simulink model "feedback_lin_p_with_noise_realistic"  (R2023a)
settings: Solver=ode4  StartTime=0.0  StopTime=10  FixedStep=0.001  RelTol=1e-3
InitFcn:
  | Init_control;
values from neighbouring files (symbols this model uses):
  ModelInit_AngEuler = [0, 0, 0]    [Init_control.m]
  ModelInit_PosE = [0, 0, 0]    [Init_control.m]
  ModelInit_Rads = 0    [Init_control.m]
  ModelInit_RateB = [0, 0, 0]    [Init_control.m]
  ModelInit_VelB = [0, 0, 0]    [Init_control.m]
  P = 0.5 * eye(6)    [Init_control.m]
  Ts = 0.002    [Init_control.m]
undefined symbols (not defined in the file or in its folder): lincontroller, ModelParam_envGravityAcc, ModelParam_motorCr, ModelParam_motorJm, ModelParam_motorT, ModelParam_motorWb, ModelParam_rotorCm, ModelParam_rotorCt, ModelParam_uavCCm, ModelParam_uavCd, ModelParam_uavJ, ModelParam_uavMass, ModelParam_uavR, quadParams
libraries: simulink x2, sharedutil x2
settings Model: Creator=wsh  LastModifiedBy=matte
settings SolverCC: AlgebraicLoopSolver=TrustRegion
settings DataIOCC: ReturnWorkspaceOutputs=off
settings DebuggingCC: UnconnectedInputMsg=warning  UnconnectedOutputMsg=warning  UnconnectedLineMsg=warning  BusObjectLabelMismatch=error  ArithmeticOperatorsInVariantConditions=warning
settings ModelReferenceCC: EnableRefExpFcnMdlSchedulingChecks=on
settings SFSimCC: SimUseLocalCustomCode=off  CustomCodeUndefinedFunction=UseInterfaceOnly
settings RTWCC: RTWUseLocalCustomCode=off
settings CodeAppCC: StateflowObjectComments=on

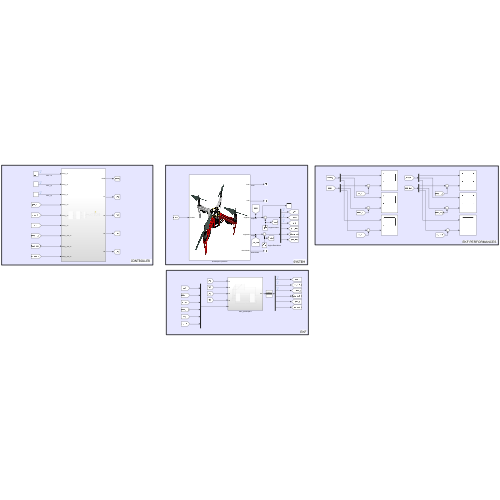
[thumbnail: Simulink's stored preview of the top-level diagram]
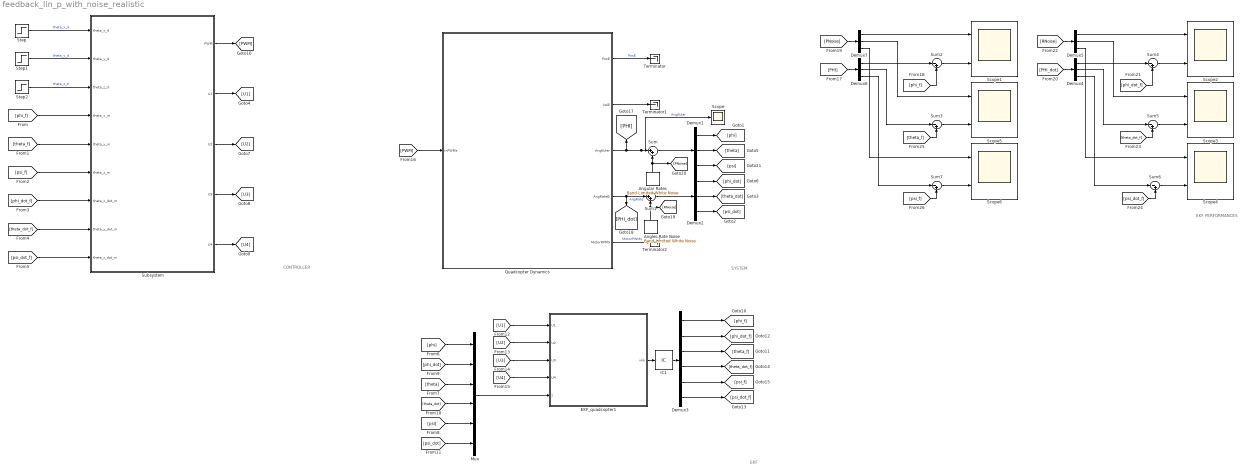
== system feedback_lin_p_with_noise_realistic ==
  note: CONTROLLER
  note: SYSTEM
  note: EKF
  note: EKF PERFORMANCES
  "Angles Rate Noise " : simulink/Sources/Band-Limited White Noise  Cov=[2.782739102258347e-06;2.718240466492716e-06;2.976654513986432e-06]  Ts=Ts  seed=[23341]
  Angular Rates : simulink/Sources/Band-Limited White Noise  Cov=[1.936548166270313e-08;1.809123162388460e-08;5.587443411059212e-06]  Ts=Ts  seed=[23341]
  Demux{1..2,4..7} (6 alike) : Demux  Outputs=3
  Demux3 : Demux  Outputs=6
  EKF_quadcopter1 : Subsystem
  IC1 : InitialCondition  Value=[0;0;0;0;0;0]
  Mux : Mux  Inputs=6
  Quadcopter Dynamics : Subsystem
      mask Display: image('./icon/F450.png');
  Scope : Scope
  Scope{1..6} (6 alike) : Scope  NumInputPorts=2
  Step : Step  After=0.25  SampleTime=0
  Step1 : Step  After=0.5  SampleTime=0
  Step2 : Step  After=0  SampleTime=0
  Subsystem : Subsystem
  Sum : Sum  Inputs=|++
  Sum1 : Sum  Inputs=|++
  Sum{2..7} (6 alike) : Sum  Inputs=|-+
  Terminator : Terminator
  Terminator1 : Terminator
  Terminator2 : Terminator
  wires:
  Step/1 -> Subsystem/1(theta_x_d)  "theta_x_d"
  Step1/1 -> Subsystem/2(theta_y_d)  "theta_y_d"
  Step2/1 -> Subsystem/3(theta_z_d)  "theta_z_d"
  [phi_f] -> Subsystem/4(theta_x_m)
  [theta_f] -> Subsystem/5(theta_y_m)
  [psi_f] -> Subsystem/6(theta_z_m)
  [phi_dot_f] -> Subsystem/7(theta_x_dot_m)
  [theta_dot_f] -> Subsystem/8(theta_y_dot_m)
  [psi_dot_f] -> Subsystem/9(theta_z_dot_m)
  Subsystem/2(U1) -> [U1]
  Subsystem/3(U2) -> [U2]
  Subsystem/4(U3) -> [U3]
  Subsystem/5(U4) -> [U4]
  Subsystem/1(PWM) -> [PWM]
  Demux5/3 -> Scope4/1
  [theta_dot_f] -> Sum5/2
  Demux5/2 -> Scope3/1
  Sum6/1 -> Scope4/2
  [PHI_dot] -> Demux4/1
  Demux4/1 -> Sum4/1
  Demux7/3 -> Scope6/1
  Demux4/2 -> Sum5/1
  Demux6/3 -> Sum7/1
  Demux6/2 -> Sum3/1
  [psi_f] -> Sum7/2
  [PNoise] -> Demux7/1
  Demux7/2 -> Scope5/1
  Sum3/1 -> Scope5/2
  [phi_f] -> Sum2/2
  Demux4/3 -> Sum6/1
  Demux7/1 -> Scope1/1
  Quadcopter Dynamics/4(AngRateB) -> Sum1/1, [PHI_dot]  "AngRate"
  [PHI] -> Demux6/1
  Demux3/2 -> [phi_dot_f]
  Quadcopter Dynamics/5(MotorRPMS) -> Terminator2/1  "MotorPWMs"
  Mux/1 -> EKF_quadcopter1/5(z)
  [psi_dot] -> Mux/6
  [U1] -> EKF_quadcopter1/1(U1)
  Sum2/1 -> Scope1/2
  [phi] -> Mux/1
  Demux6/1 -> Sum2/1
  [U2] -> EKF_quadcopter1/2(U2)
  [RNoise] -> Demux5/1
  Demux2/2 -> [theta_dot]
  [theta] -> Mux/3
  [psi] -> Mux/5
  Sum1/1 -> Demux2/1
  [phi_dot] -> Mux/2
  Angular Rates/1 -> [PNoise], Sum/2
  Demux2/1 -> [phi_dot]
  [U3] -> EKF_quadcopter1/3(U3)
  [theta_f] -> Sum3/2
  Demux1/3 -> [psi]
  [theta_dot] -> Mux/4
  [phi_dot_f] -> Sum4/2
  Sum/1 -> Demux1/1
  IC1/1 -> Demux3/1
  Demux3/3 -> [theta_f]
  Sum4/1 -> Scope2/2
  Demux3/5 -> [psi_f]
  Quadcopter Dynamics/1(PosE) -> Terminator/1  "PosE"
  Demux3/4 -> [theta_dot_f]
  Demux1/2 -> [theta]
  Demux2/3 -> [psi_dot]
  Demux1/1 -> [phi]
  Quadcopter Dynamics/2(VelE) -> Terminator1/1
  Quadcopter Dynamics/3(AngEuler) -> Scope/1, Sum/1, [PHI]  "AngEular"
  [U4] -> EKF_quadcopter1/4(U4)
  Demux3/6 -> [psi_dot_f]
  Sum5/1 -> Scope3/2
  "Angles Rate Noise "/1 -> [RNoise], Sum1/2
  Demux5/1 -> Scope2/1
  [psi_dot_f] -> Sum6/2
  Demux3/1 -> [phi_f]
  [PWM] -> Quadcopter Dynamics/1(inPWMs)
  Sum7/1 -> Scope6/2
  EKF_quadcopter1/1(xkk) -> IC1/1

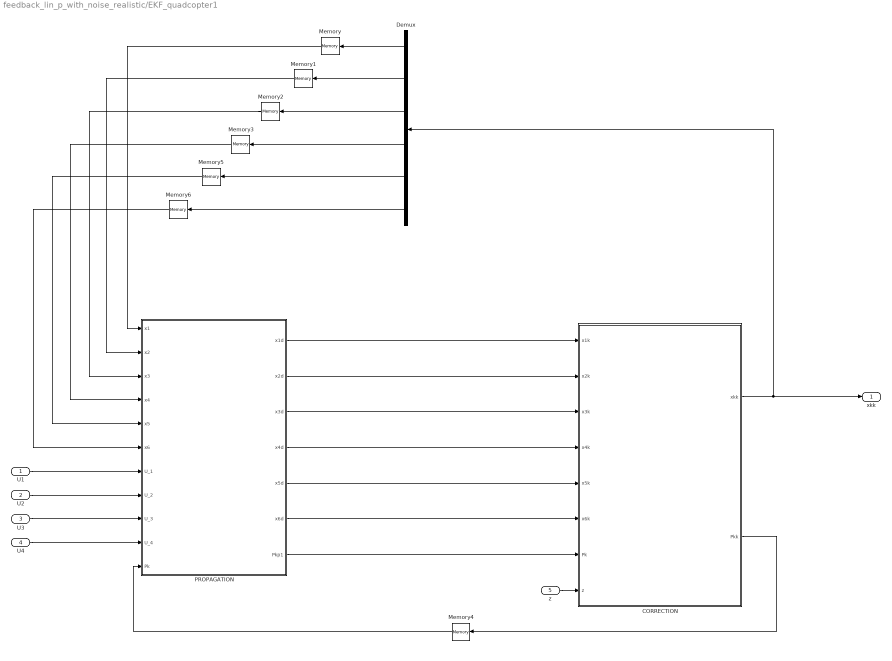
== system feedback_lin_p_with_noise_realistic/EKF_quadcopter1 ==
  U1 : Inport
  U2 : Inport  Port=2
  U3 : Inport  Port=3
  U4 : Inport  Port=4
  z : Inport  Port=5
  CORRECTION : MATLAB Function  TreatAsAtomicUnit=on
  Demux : Demux  Outputs=6
  Memory{,1..3,5..6} (6 alike) : Memory
  Memory4 : Memory  InitialCondition=P
  PROPAGATION : MATLAB Function  TreatAsAtomicUnit=on
  xkk : Outport
  wires:
  PROPAGATION/1(x1d) -> CORRECTION/1(x1k)
  PROPAGATION/2(x2d) -> CORRECTION/2(x2k)
  PROPAGATION/3(x3d) -> CORRECTION/3(x3k)
  PROPAGATION/4(x4d) -> CORRECTION/4(x4k)
  Memory4/1 -> PROPAGATION/11(Pk)
  U1/1 -> PROPAGATION/7(U_1)
  U2/1 -> PROPAGATION/8(U_2)
  U3/1 -> PROPAGATION/9(U_3)
  U4/1 -> PROPAGATION/10(U_4)
  PROPAGATION/7(Pkp1) -> CORRECTION/7(Pk)
  CORRECTION/2(Pkk) -> Memory4/1
  z/1 -> CORRECTION/8(z)
  Demux/1 -> Memory/1
  Demux/2 -> Memory1/1
  Demux/3 -> Memory2/1
  Demux/4 -> Memory3/1
  CORRECTION/1(xkk) -> Demux/1, xkk/1
  Memory/1 -> PROPAGATION/1(x1)
  Memory1/1 -> PROPAGATION/2(x2)
  Memory2/1 -> PROPAGATION/3(x3)
  Memory3/1 -> PROPAGATION/4(x4)
  PROPAGATION/6(x6d) -> CORRECTION/6(x6k)
  PROPAGATION/5(x5d) -> CORRECTION/5(x5k)
  Demux/5 -> Memory5/1
  Memory5/1 -> PROPAGATION/5(x5)
  Demux/6 -> Memory6/1
  Memory6/1 -> PROPAGATION/6(x6)

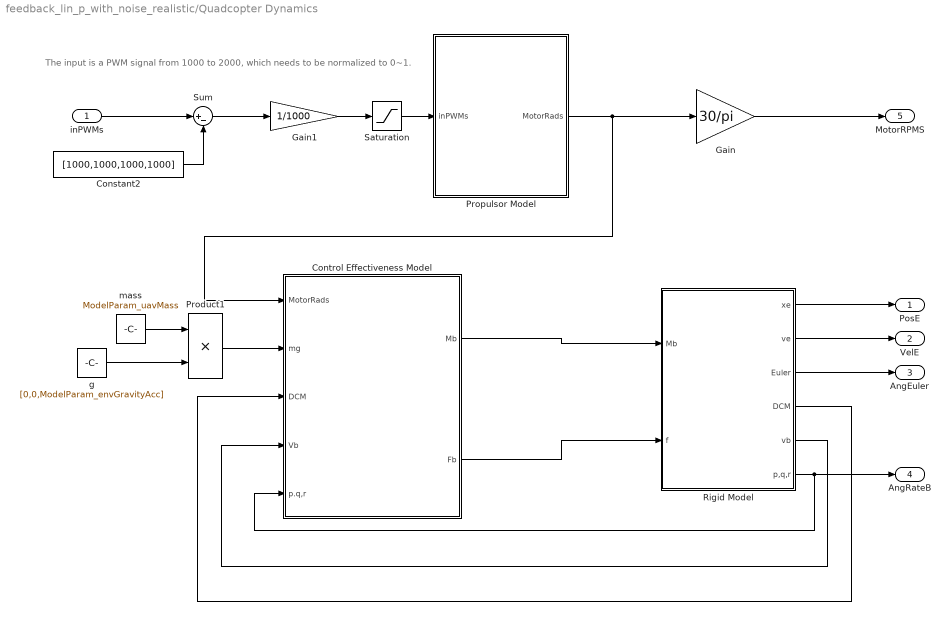
== system feedback_lin_p_with_noise_realistic/Quadcopter Dynamics ==
  note: The input is a PWM signal from 1000 to 2000,
      | which needs to be normalized to 0~1.
  inPWMs : Inport
  Constant2 : Constant  Value=[1000,1000,1000,1000]
  Control Effectiveness Model : Subsystem
  Gain : Gain  Gain=30/pi
  Gain1 : Gain  Gain=1/1000
  Product1 : Product
  Propulsor Model : Subsystem
  Rigid Model : Subsystem
  Saturation : Saturate  UpperLimit=1  LowerLimit=0
  Sum : Sum  Inputs=|+-
  g : Constant  Value=[0,0,ModelParam_envGravityAcc]
  mass : Constant  Value=ModelParam_uavMass
  PosE : Outport  VectorParamsAs1DForOutWhenUnconnected=off
  VelE : Outport  Port=2  VectorParamsAs1DForOutWhenUnconnected=off
  AngEuler : Outport  Port=3  VectorParamsAs1DForOutWhenUnconnected=off
  AngRateB : Outport  Port=4  VectorParamsAs1DForOutWhenUnconnected=off
  MotorRPMS : Outport  Port=5  VectorParamsAs1DForOutWhenUnconnected=off
  wires:
  Saturation/1 -> Propulsor Model/1(inPWMs)
  Rigid Model/6("p,q,r ") -> Control Effectiveness Model/5(p.q,r), AngRateB/1
  mass/1 -> Product1/1
  Rigid Model/4(DCM) -> Control Effectiveness Model/3(DCM)
  Propulsor Model/1(MotorRads) -> Gain/1, Control Effectiveness Model/1(MotorRads)
  Gain1/1 -> Saturation/1
  Rigid Model/2(ve) -> VelE/1
  Sum/1 -> Gain1/1
  Product1/1 -> Control Effectiveness Model/2(mg)
  Rigid Model/5("vb ") -> Control Effectiveness Model/4(Vb)
  Rigid Model/1("xe ") -> PosE/1
  Rigid Model/3(Euler) -> AngEuler/1
  Control Effectiveness Model/1(Mb) -> Rigid Model/1(Mb)
  inPWMs/1 -> Sum/1
  Control Effectiveness Model/2(Fb) -> Rigid Model/2(f)
  Constant2/1 -> Sum/2
  g/1 -> Product1/2
  Gain/1 -> MotorRPMS/1

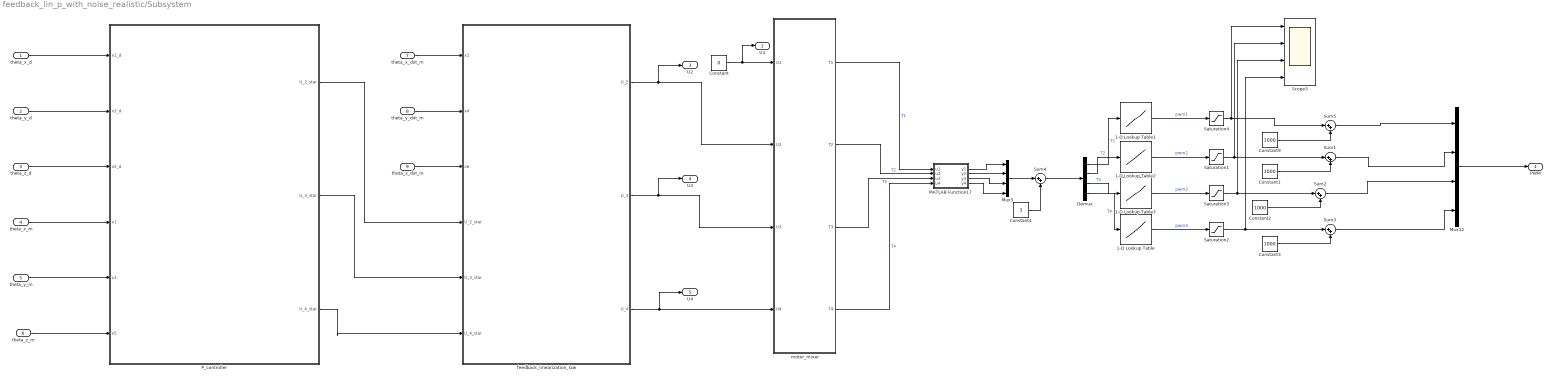
== system feedback_lin_p_with_noise_realistic/Subsystem ==
  theta_x_d : Inport
  theta_y_d : Inport  Port=2
  theta_z_d : Inport  Port=3
  theta_x_m : Inport  Port=4
  theta_y_m : Inport  Port=5
  theta_z_m : Inport  Port=6
  theta_x_dot_m : Inport  Port=7
  theta_y_dot_m : Inport  Port=8
  theta_z_dot_m : Inport  Port=9
  1-D Lookup Table : Lookup_n-D  NumberOfTableDimensions=1  BreakpointsForDimension1=[0;0.06477642396;0.16;0.63;2.44;4.43;6.92;8.77;10.52;11.63;12.03;12.09;12.091;12.092;12.093;12.094;12.095;12.096;12.097;12.098;12.099]  Table=[0;50;100;150;200;250;300;350;400;450;500;550;600;650;700;750;800;850;900;950;1000]  InternalRulePriority=Speed  RndMeth=Simplest
  1-D Lookup Table1 : Lookup_n-D  NumberOfTableDimensions=1  BreakpointsForDimension1=[0;0.02;0.06;0.29;0.73;1.07;1.88;2.91;4;5.06;6.71;7.86;9.41;10.86;11.45;11.82;12.07;12.31;12.52;12.74;12.75]  Table=[0;50;100;150;200;250;300;350;400;450;500;550;600;650;700;750;800;850;900;950;1000]  InternalRulePriority=Speed  RndMeth=Simplest
  1-D Lookup Table2 : Lookup_n-D  NumberOfTableDimensions=1  BreakpointsForDimension1=[0;0.05;0.39;1.67;3.19;5.57;8.07;10.01;10.71;11.06;11.42;11.53;11.55;11.551;11.552;11.553;11.554;11.555;11.556;11.557;11.558]  Table=[0;50;100;150;200;250;300;350;400;450;500;550;600;650;700;750;800;850;900;950;1000]  InternalRulePriority=Speed  RndMeth=Simplest
  1-D Lookup Table3 : Lookup_n-D  NumberOfTableDimensions=1  BreakpointsForDimension1=[0;0.06;0.23;0.89;2.47;3.9;5.86;7.81;9.42;10.12;10.6;11.01;11.34;11.39;11.391;11.392;11.393;11.394;11.395;11.396;11.397]  Table=[0;50;100;150;200;250;300;350;400;450;500;550;600;650;700;750;800;850;900;950;1000]  InternalRulePriority=Speed  RndMeth=Simplest
  Constant : Constant  Value=0
  Constant{1..3,9} (4 alike) : Constant  Value=1000  SampleTime=-1
  Constant4 : Constant  Value=3
  Demux : Demux
  MATLAB Function17 : MATLAB Function  TreatAsAtomicUnit=on
  Mux12 : Mux
  Mux5 : Mux
  P_controller : MATLAB Function  TreatAsAtomicUnit=on
  Saturation{1..4} (4 alike) : Saturate  UpperLimit=1000  LowerLimit=0
  Scope3 : Scope  NumInputPorts=4
  Sum{1..5} (5 alike) : Sum  Inputs=|++
  feedback_linearization_law : MATLAB Function  TreatAsAtomicUnit=on
  motor_mixer : MATLAB Function  SystemSampleTime=0.004
  PWM : Outport  VectorParamsAs1DForOutWhenUnconnected=off
  U1 : Outport  Port=2
  U2 : Outport  Port=3
  U3 : Outport  Port=4
  U4 : Outport  Port=5
  wires:
  theta_x_d/1 -> P_controller/1(x1_d)
  theta_y_d/1 -> P_controller/2(x3_d)
  theta_z_d/1 -> P_controller/3(x5_d)
  theta_x_m/1 -> P_controller/4(x1)
  theta_y_m/1 -> P_controller/5(x3)
  theta_z_m/1 -> P_controller/6(x5)
  Mux12/1 -> PWM/1
  motor_mixer/4(T4) -> MATLAB Function17/4(u4)  "T4"
  1-D Lookup Table3/1 -> Saturation3/1  "pwm3"
  motor_mixer/1(T1) -> MATLAB Function17/1(u1)  "T1"
  motor_mixer/3(T3) -> MATLAB Function17/3(u3)  "T3"
  1-D Lookup Table2/1 -> Saturation1/1  "pwm2"
  1-D Lookup Table1/1 -> Saturation4/1  "pwm1"
  motor_mixer/2(T2) -> MATLAB Function17/2(u2)  "T2"
  Sum5/1 -> Mux12/1
  Saturation4/1 -> Scope3/1, Sum5/1
  Constant9/1 -> Sum5/2
  1-D Lookup Table/1 -> Saturation2/1  "pwm4"
  Saturation1/1 -> Scope3/2, Sum1/1
  Sum1/1 -> Mux12/2
  Constant1/1 -> Sum1/2
  Saturation3/1 -> Scope3/3, Sum2/1
  Sum2/1 -> Mux12/3
  Constant2/1 -> Sum2/2
  Saturation2/1 -> Scope3/4, Sum3/1
  Sum3/1 -> Mux12/4
  Constant3/1 -> Sum3/2
  P_controller/1(U_2_star) -> feedback_linearization_law/4(U_2_star)
  Constant4/1 -> Sum4/2
  Demux/3 -> 1-D Lookup Table3/1  "T3"
  Sum4/1 -> Demux/1
  Mux5/1 -> Sum4/1
  MATLAB Function17/3(y3) -> Mux5/3
  MATLAB Function17/1(y1) -> Mux5/1
  MATLAB Function17/4(y4) -> Mux5/4
  Demux/4 -> 1-D Lookup Table/1  "T4"
  MATLAB Function17/2(y2) -> Mux5/2
  Demux/2 -> 1-D Lookup Table2/1  "T2"
  Demux/1 -> 1-D Lookup Table1/1  "T1"
  feedback_linearization_law/1(U_2) -> U2/1, motor_mixer/2(U2)
  feedback_linearization_law/2(U_3) -> U3/1, motor_mixer/3(U3)
  feedback_linearization_law/3(U_4) -> U4/1, motor_mixer/4(U4)
  P_controller/2(U_3_star) -> feedback_linearization_law/5(U_3_star)
  P_controller/3(U_4_star) -> feedback_linearization_law/6(U_4_star)
  Constant/1 -> U1/1, motor_mixer/1(U1)
  theta_x_dot_m/1 -> feedback_linearization_law/1(x2)
  theta_y_dot_m/1 -> feedback_linearization_law/2(x4)
  theta_z_dot_m/1 -> feedback_linearization_law/3(x6)

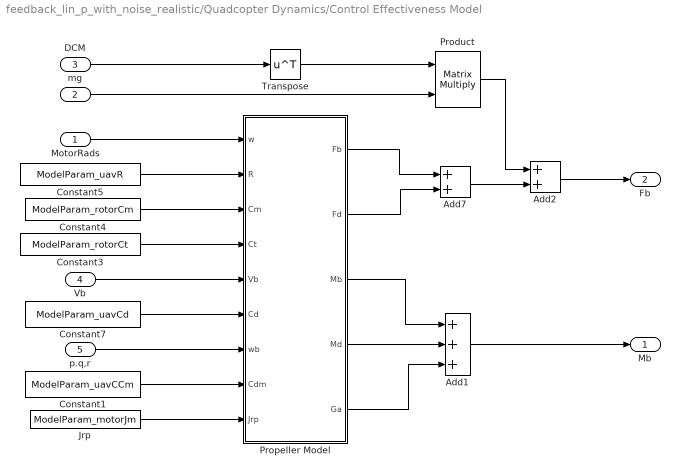
== system feedback_lin_p_with_noise_realistic/Quadcopter Dynamics/Control Effectiveness Model ==
  MotorRads : Inport
  mg : Inport  Port=2
  DCM : Inport  Port=3
  Vb : Inport  Port=4
  p.q,r : Inport  Port=5
  Add1 : Sum  Inputs=+++
  Add2 : Sum
  Add7 : Sum
  Constant1 : Constant  Value=ModelParam_uavCCm
  Constant3 : Constant  Value=ModelParam_rotorCt
  Constant4 : Constant  Value=ModelParam_rotorCm
  Constant5 : Constant  Value=ModelParam_uavR
  Constant7 : Constant  Value=ModelParam_uavCd
  Jrp : Constant  Value=ModelParam_motorJm
  Product : Product  Multiplication=Matrix(*)
  Propeller Model : MATLAB Function  TreatAsAtomicUnit=on
  Transpose : Math  Operator=transpose  SignedPower=on
  Mb : Outport  VectorParamsAs1DForOutWhenUnconnected=off
  Fb : Outport  Port=2  VectorParamsAs1DForOutWhenUnconnected=off
  wires:
  Add2/1 -> Fb/1
  Constant3/1 -> Propeller Model/4(Ct)
  Propeller Model/2(Fd) -> Add7/2
  Add7/1 -> Add2/2
  Propeller Model/1(Fb) -> Add7/1
  Product/1 -> Add2/1
  mg/1 -> Product/2
  DCM/1 -> Transpose/1
  Constant7/1 -> Propeller Model/6(Cd)
  Vb/1 -> Propeller Model/5(Vb)
  Constant5/1 -> Propeller Model/2(R)
  Constant4/1 -> Propeller Model/3(Cm)
  MotorRads/1 -> Propeller Model/1(w)
  Transpose/1 -> Product/1
  Propeller Model/3(Mb) -> Add1/1
  Propeller Model/4(Md) -> Add1/2
  Add1/1 -> Mb/1
  p.q,r/1 -> Propeller Model/7(wb)
  Constant1/1 -> Propeller Model/8(Cdm)
  Jrp/1 -> Propeller Model/9(Jrp)
  Propeller Model/5(Ga) -> Add1/3

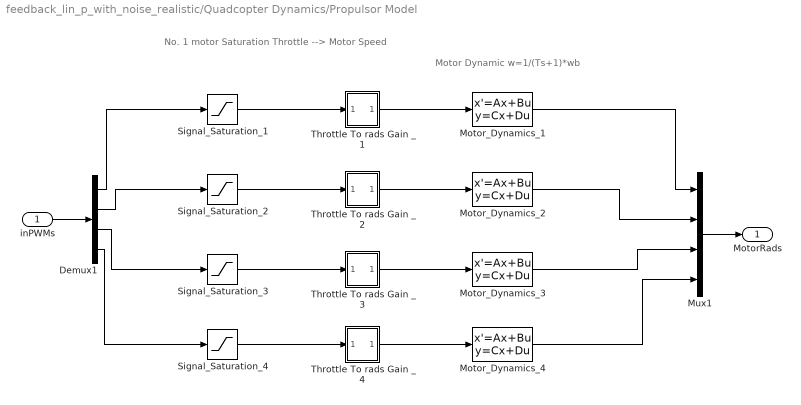
== system feedback_lin_p_with_noise_realistic/Quadcopter Dynamics/Propulsor Model ==
  note: Motor Dynamic
      | w=1/(Ts+1)*wb
  note: No. 1 motor
      |
      |          Saturation             Throttle --> Motor Speed
  inPWMs : Inport
  Demux1 : Demux
  Motor_Dynamics_{1..4} (4 alike) : StateSpace  A=-1/ModelParam_motorT  C=1/ModelParam_motorT  D=0  InitialCondition=ModelInit_Rads*ModelParam_motorT
  Mux1 : Mux
  Signal_Saturation_{1..4} (4 alike) : Saturate  UpperLimit=1  LowerLimit=0
  Throttle To rads Gain _1 : Subsystem
  Throttle To rads Gain _2 : Subsystem
  Throttle To rads Gain _3 : Subsystem
  Throttle To rads Gain _4 : Subsystem
  MotorRads : Outport  VectorParamsAs1DForOutWhenUnconnected=off
  wires:
  Throttle To rads Gain _4/1(Out5) -> Motor_Dynamics_4/1
  Signal_Saturation_4/1 -> Throttle To rads Gain _4/1(In5)
  Signal_Saturation_3/1 -> Throttle To rads Gain _3/1(In5)
  Signal_Saturation_2/1 -> Throttle To rads Gain _2/1(In5)
  Motor_Dynamics_4/1 -> Mux1/4
  Motor_Dynamics_3/1 -> Mux1/3
  Motor_Dynamics_2/1 -> Mux1/2
  Motor_Dynamics_1/1 -> Mux1/1
  Signal_Saturation_1/1 -> Throttle To rads Gain _1/1(In5)
  Mux1/1 -> MotorRads/1
  Throttle To rads Gain _3/1(Out5) -> Motor_Dynamics_3/1
  Throttle To rads Gain _2/1(Out5) -> Motor_Dynamics_2/1
  Throttle To rads Gain _1/1(Out5) -> Motor_Dynamics_1/1
  inPWMs/1 -> Demux1/1
  Demux1/4 -> Signal_Saturation_4/1
  Demux1/3 -> Signal_Saturation_3/1
  Demux1/2 -> Signal_Saturation_2/1
  Demux1/1 -> Signal_Saturation_1/1

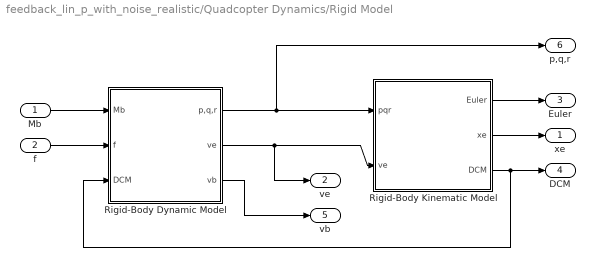
== system feedback_lin_p_with_noise_realistic/Quadcopter Dynamics/Rigid Model ==
  Mb : Inport
  f : Inport  Port=2
  Rigid-Body Dynamic Model : Subsystem
  "Rigid-Body Kinematic Model " : Subsystem
  "xe " : Outport  VectorParamsAs1DForOutWhenUnconnected=off
  ve : Outport  Port=2  VectorParamsAs1DForOutWhenUnconnected=off
  Euler : Outport  Port=3  VectorParamsAs1DForOutWhenUnconnected=off
  DCM : Outport  Port=4  VectorParamsAs1DForOutWhenUnconnected=off
  "vb " : Outport  Port=5  VectorParamsAs1DForOutWhenUnconnected=off
  "p,q,r " : Outport  Port=6  VectorParamsAs1DForOutWhenUnconnected=off
  wires:
  Rigid-Body Dynamic Model/1("p,q,r ") -> "Rigid-Body Kinematic Model "/1(pqr), "p,q,r "/1
  "Rigid-Body Kinematic Model "/1(Euler) -> Euler/1
  "Rigid-Body Kinematic Model "/3(DCM) -> Rigid-Body Dynamic Model/3(DCM), DCM/1
  Mb/1 -> Rigid-Body Dynamic Model/1(Mb)
  f/1 -> Rigid-Body Dynamic Model/2(f)
  Rigid-Body Dynamic Model/2(ve) -> "Rigid-Body Kinematic Model "/2(ve), ve/1
  Rigid-Body Dynamic Model/3("vb ") -> "vb "/1
  "Rigid-Body Kinematic Model "/2("xe ") -> "xe "/1

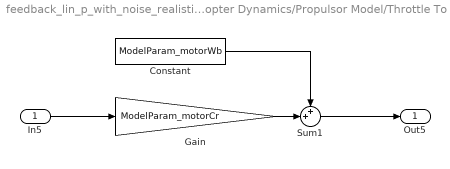
== system feedback_lin_p_with_noise_realistic/Quadcopter Dynamics/Propulsor Model/Throttle To rads Gain _1 ==
  In5 : Inport
  Constant : Constant  Value=ModelParam_motorWb
  Gain : Gain  Gain=ModelParam_motorCr
  Sum1 : Sum  Inputs=++|
  Out5 : Outport  VectorParamsAs1DForOutWhenUnconnected=off
  wires:
  Constant/1 -> Sum1/1
  Gain/1 -> Sum1/2
  In5/1 -> Gain/1
  Sum1/1 -> Out5/1

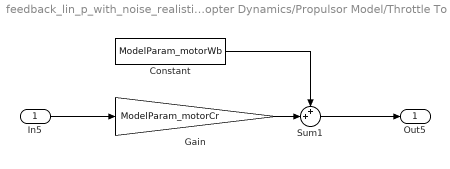
== system feedback_lin_p_with_noise_realistic/Quadcopter Dynamics/Propulsor Model/Throttle To rads Gain _2 ==
  In5 : Inport
  Constant : Constant  Value=ModelParam_motorWb
  Gain : Gain  Gain=ModelParam_motorCr
  Sum1 : Sum  Inputs=++|
  Out5 : Outport  VectorParamsAs1DForOutWhenUnconnected=off
  wires:
  Sum1/1 -> Out5/1
  In5/1 -> Gain/1
  Gain/1 -> Sum1/2
  Constant/1 -> Sum1/1

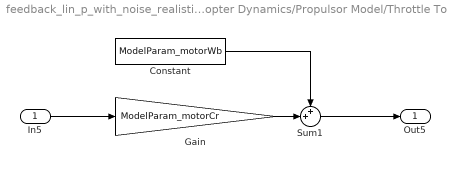
== system feedback_lin_p_with_noise_realistic/Quadcopter Dynamics/Propulsor Model/Throttle To rads Gain _3 ==
  In5 : Inport
  Constant : Constant  Value=ModelParam_motorWb
  Gain : Gain  Gain=ModelParam_motorCr
  Sum1 : Sum  Inputs=++|
  Out5 : Outport  VectorParamsAs1DForOutWhenUnconnected=off
  wires:
  Constant/1 -> Sum1/1
  Gain/1 -> Sum1/2
  In5/1 -> Gain/1
  Sum1/1 -> Out5/1

== system feedback_lin_p_with_noise_realistic/Quadcopter Dynamics/Propulsor Model/Throttle To rads Gain _4 ==
  In5 : Inport
  Constant : Constant  Value=ModelParam_motorWb
  Gain : Gain  Gain=ModelParam_motorCr
  Sum1 : Sum  Inputs=++|
  Out5 : Outport  VectorParamsAs1DForOutWhenUnconnected=off
  wires:
  Sum1/1 -> Out5/1
  In5/1 -> Gain/1
  Gain/1 -> Sum1/2
  Constant/1 -> Sum1/1

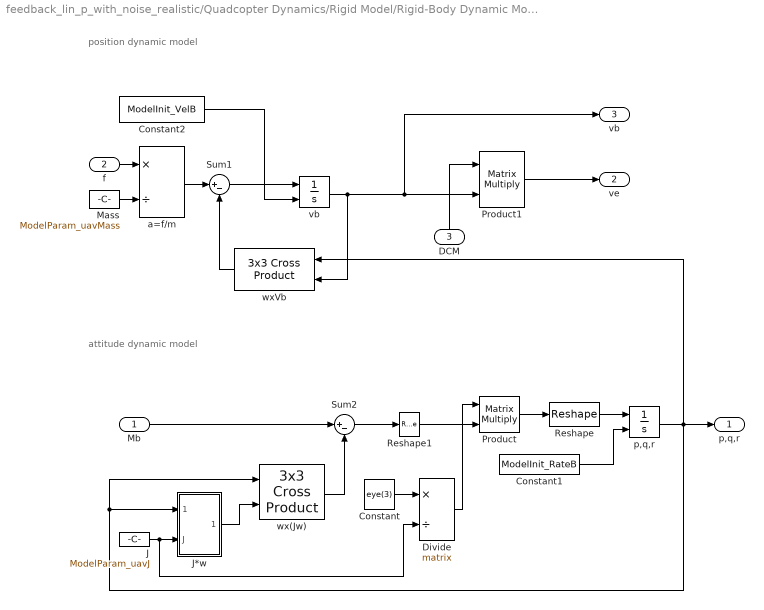
== system feedback_lin_p_with_noise_realistic/Quadcopter Dynamics/Rigid Model/Rigid-Body Dynamic Model ==
  note: attitude dynamic model
  note: position dynamic model
  Mb : Inport
  f : Inport  Port=2
  DCM : Inport  Port=3
  " Mass " : Constant  Value=ModelParam_uavMass
  Constant : Constant  Value=eye(3)
  Constant1 : Constant  Value=ModelInit_RateB
  Constant2 : Constant  Value=ModelInit_VelB
  Divide : Product  Inputs=*/  Multiplication=Matrix(*)
  "J " : Constant  Value=ModelParam_uavJ
  J*w : Subsystem
  Product : Product  Multiplication=Matrix(*)
  Product1 : Product  Multiplication=Matrix(*)
  Reshape : Reshape  OutputDimensionality=Customize  OutputDimensions=[3,1]
  Reshape1 : Reshape  OutputDimensionality=Column vector (2-D)
  Sum1 : Sum  Inputs=|+-
  Sum2 : Sum  Inputs=|+-
  a=f/m : Product  Inputs=*/
  p,q,r : Integrator  InitialConditionSource=external
  vb : Integrator  InitialConditionSource=external
  wx(Jw) : sharedutil/3x3 Cross Product  aMode=aMode
  wxVb : sharedutil/3x3 Cross Product  aMode=aMode
  "p,q,r " : Outport  VectorParamsAs1DForOutWhenUnconnected=off
  ve : Outport  Port=2  VectorParamsAs1DForOutWhenUnconnected=off
  "vb " : Outport  Port=3  VectorParamsAs1DForOutWhenUnconnected=off
  wires:
  Product/1 -> Reshape/1
  Reshape1/1 -> Product/2
  Constant/1 -> Divide/1
  Divide/1 -> Product/1
  Sum2/1 -> Reshape1/1
  "J "/1 -> Divide/2, J*w/2(J)
  p,q,r/1 -> "p,q,r "/1, J*w/1(p q r), wx(Jw)/1, wxVb/1
  J*w/1("J*w ") -> wx(Jw)/2
  Mb/1 -> Sum2/1
  wx(Jw)/1 -> Sum2/2
  Constant2/1 -> vb/2
  f/1 -> a=f/m/1
  Product1/1 -> ve/1
  wxVb/1 -> Sum1/2
  a=f/m/1 -> Sum1/1
  Sum1/1 -> vb/1
  vb/1 -> Product1/2, "vb "/1, wxVb/2
  " Mass "/1 -> a=f/m/2
  DCM/1 -> Product1/1
  Reshape/1 -> p,q,r/1
  Constant1/1 -> p,q,r/2

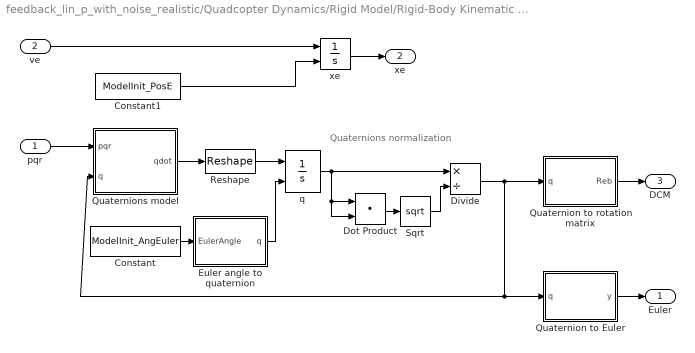
== system feedback_lin_p_with_noise_realistic/Quadcopter Dynamics/Rigid Model/Rigid-Body Kinematic Model  ==
  note: Quaternions
      | normalization
  pqr : Inport
  ve : Inport  Port=2
  Constant : Constant  Value=ModelInit_AngEuler
  Constant1 : Constant  Value=ModelInit_PosE
  Divide : Product  Inputs=*/
  Dot Product : DotProduct  OutDataTypeStr=Inherit: Inherit via internal rule
  Euler angle to quaternion : MATLAB Function
  Quaternion to Euler : MATLAB Function
  Quaternion to rotation matrix : MATLAB Function
  Quaternions model : MATLAB Function  TreatAsAtomicUnit=on
  Reshape : Reshape  OutputDimensionality=Customize  OutputDimensions=[4,1]
  Sqrt : Sqrt
  q : Integrator  InitialConditionSource=external
  xe : Integrator  InitialConditionSource=external
  Euler : Outport  VectorParamsAs1DForOutWhenUnconnected=off
  "xe " : Outport  Port=2  VectorParamsAs1DForOutWhenUnconnected=off
  DCM : Outport  Port=3  VectorParamsAs1DForOutWhenUnconnected=off
  wires:
  Divide/1 -> Quaternion to rotation matrix/1(q), Quaternions model/2(q), Quaternion to Euler/1(q)
  Dot Product/1 -> Sqrt/1
  pqr/1 -> Quaternions model/1(pqr)
  q/1 -> Divide/1, Dot Product/1, Dot Product/2
  Quaternions model/1(qdot) -> Reshape/1
  Quaternion to rotation matrix/1(Reb) -> DCM/1
  Quaternion to Euler/1(y) -> Euler/1
  Constant/1 -> Euler angle to quaternion/1(EulerAngle)
  Euler angle to quaternion/1(q) -> q/2
  Reshape/1 -> q/1
  ve/1 -> xe/1
  xe/1 -> "xe "/1
  Constant1/1 -> xe/2
  Sqrt/1 -> Divide/2

== system feedback_lin_p_with_noise_realistic/Quadcopter Dynamics/Rigid Model/Rigid-Body Dynamic Model/J*w ==
  p q r : Inport
  J : Inport  Port=2
  J*w : Product  Multiplication=Matrix(*)
  "J*w " : Outport  VectorParamsAs1DForOutWhenUnconnected=off
  wires:
  J*w/1 -> "J*w "/1
  J/1 -> J*w/1
  p q r/1 -> J*w/2

== matlab function feedback_lin_p_with_noise_realistic/Quadcopter Dynamics/Rigid Model/Rigid-Body Kinematic Model /Quaternion to Euler ==
  data: q input; y output
function y = fcn(q)
 %Function description:
%  Quaternions to Euler
phi = atan2(2*(q(1)*q(2) + q(3)*q(4)), (1 - 2*(q(2)*q(2) + q(3)*q(3))));
theta = asin(2*(q(1)*q(3) - q(2)*q(4)));
psi = atan2(2*(q(1)*q(4) + q(2)*q(3)), (1 - 2*(q(3)*q(3) + q(4)*q(4))));
y = [phi theta psi];

== matlab function feedback_lin_p_with_noise_realistic/Quadcopter Dynamics/Rigid Model/Rigid-Body Kinematic Model /Quaternions model ==
  data: pqr input; qdot output; q input
function qdot = fcn(pqr, q)
%Function description:
%  Quaternions model
qdot = 0.5*[0, -pqr(1), -pqr(2), -pqr(3); pqr(1), 0, pqr(3), -pqr(2); pqr(2), -pqr(3), 0, pqr(1); pqr(3), pqr(2), -pqr(1), 0]*q;

== matlab function feedback_lin_p_with_noise_realistic/Quadcopter Dynamics/Rigid Model/Rigid-Body Kinematic Model /Euler angle to quaternion ==
  data: EulerAngle input; q output
function q = fcn(EulerAngle)
%Function description:
%  Get quaternions from Euler angle
q0 =  cos(EulerAngle(1)/2)*cos(EulerAngle(2)/2)*cos(EulerAngle(3)/2) + sin(EulerAngle(1)/2)*sin((EulerAngle(2)/2))*sin((EulerAngle(3)/2));
q1 = sin(EulerAngle(1)/2)*cos(EulerAngle(2)/2)*cos(EulerAngle(3)/2) - cos(EulerAngle(1)/2)*sin((EulerAngle(2)/2))*sin((EulerAngle(3)/2));
q2 = cos(EulerAngle(1)/2)*sin(EulerAngle(2)/2)*cos(EulerAngle(3)/2) + sin(EulerAngle(1)/2)*cos((EulerAngle(2)/2))*sin((EulerAngle(3)/2));
q3 = cos(EulerAngle(1)/2)*cos(EulerAngle(2)/2)*sin(EulerAngle(3)/2) - sin(EulerAngle(1)/2)*sin((EulerAngle(2)/2))*cos((EulerAngle(3)/2));
q = [q0 q1 q2 q3]';

== matlab function feedback_lin_p_with_noise_realistic/Quadcopter Dynamics/Control Effectiveness Model/Propeller Model ==
  data: w input; R input; Fb output; Fd output; Mb output; Cm input; Ct input; Vb input; Cd input; wb input; Md output; Cdm input; Jrp input; Ga output
function [Fb, Fd, Mb, Md, Ga] = fcn(w, R, Cm, Ct, Vb, Cd,wb, Cdm, Jrp)
 %Function description:
 %  Obtain the force and torque acting on the body. The airframe of the
 %  quadrotor is as follows:
 %3↓   1↑
 %  \ /
 %  / \
 %2↑   4↓
 %↑ stands for counterclockwise and ↓stands for clockwise.
 %Input：
 %  w: motor speed，unit：rad/s
 %  R: body radius(m)
 %  Cm: torque coefficient
 %  Ct: thrust coefficient
 %  Vb: aircraft speed in the body coordinate system
 %  Cd: damping coefficient
 %  wb: angular velocity in the body coordinate system
 %  Cdm: damping moment coefficient vector
 %  Jrp:  moment of inertia of motor rotor + propeller
 %Output:
 %  Fb: thrust under the body coordinate system
 %  Fd: aerodynamic force under the body coordinate system
 %  Mb: torque under the body coordinate system
 %  Md: aerodynamic moment
 %  Ga: gyro moment
 M_rctcm = [-sin(pi/4)*R*Ct, sin(pi/4)*R*Ct, sin(pi/4)*R*Ct, -sin(pi/4)*R*Ct;
            sin(pi/4)*R*Ct, -sin(pi/4)*R*Ct, sin(pi/4)*R*Ct, -sin(pi/4)*R*Ct;
            Cm, Cm, -Cm, -Cm];
 Mb = M_rctcm*(w.^2);  % torque
 
 Fb = [0; 0; -sum(Ct*(w.^2))];  % thrust
 Fd = -Cd*Vb.*abs(Vb)*0.5;  % aerodynamic force
 Md = -Cdm.*wb.*abs(wb);  % aerodynamic moment
 % gyro moment
 Ga = zeros(3,1);
 Ga(1) = Jrp*wb(2)*( w(1) + w(2) - w(3) - w(4));
 Ga(2) = Jrp*wb(1)*(-w(1) - w(2) + w(3) + w(4));
end

== matlab function feedback_lin_p_with_noise_realistic/Subsystem/motor_mixer ==
  data: U1 input; T1 output; U2 input; U3 input; U4 input; T2 output; T3 output; T4 output; quadParams parameter
function [T1,T2,T3,T4] = motor_mixer(U1,U2,U3,U4,quadParams)
%Function description:
%  Control allocation. The quadrotor type is X-configuration,
%  and the airframe is as follows:
%3↓   1↑
 %  \ /
 %  / \
 %2↑   4↓


% |U1|    |       1             1           1            1       |  |T1|
% |U2|  = | -L*sqrt(2)/2  L*sqrt(2)/2  L*sqrt(2)/2  -L*sqrt(2)/2 |  |T2|
% |U3|    | L*sqrt(2)/2  -L*sqrt(2)/2  L*sqrt(2)/2  -L*sqrt(2)/2 |  |T3| 
% |U4|    | kd/kt            kd/kt       -kd/kt       -kd/kt     |  |T4|



% we need to invert this in order to obtain 
% |T1|                              |U1|
% |T2| =  quadParams.MotorMixer *   |U2|
% |T3|                              |U3|
% |T4|                              |U4|

U=[U1;U2;U3;U4];
T=quadParams.MotorMixer*U;
T1=T(1);
T2=T(2);
T3=T(3);
T4=T(4);

== matlab function feedback_lin_p_with_noise_realistic/Subsystem/MATLAB Function17 ==
  data: u1 input; y1 output; u2 input; u3 input; u4 input; y2 output; y3 output; y4 output
function [y1,y2,y3,y4] = fcn(u1,u2,u3,u4)

if u1 < 0
    u2 = u2 + abs(u1);
    u1 = u1+abs(u1);
end
if u2 < 0
    u2 = u2 + abs(u2);
    u1 = u1 + abs(u2);
end
if u3 < 0
    u3 = u3 + abs(u3);
    u4 = u4 + abs(u3);
end    
if u4 < 0
    u4 = u4 + abs(u4);
    u3 = u3 + abs(u4);
end
 y1 = u1;
 y2 = u2;
 y3 = u3;
 y4 = u4;

== matlab function feedback_lin_p_with_noise_realistic/Subsystem/P_controller ==
  data: x1_d input; U_2_star output; x3_d input; x5_d input; x1 input; x3 input; x5 input; U_3_star output; U_4_star output; lincontroller parameter; quadParams parameter
function [U_2_star,U_3_star,U_4_star] = P_controller(x1_d,x3_d,x5_d,x1,x3,x5,lincontroller,quadParams)



a1=(quadParams.Jy-quadParams.Jz)/quadParams.Jx;
a2=-quadParams.Jr/quadParams.Jx;
a3=(quadParams.Jz-quadParams.Jx)/quadParams.Jy;
a4=quadParams.Jr/quadParams.Jy;
a5=(quadParams.Jx-quadParams.Jy)/quadParams.Jz;
b1=quadParams.L/quadParams.Jx;
b2=quadParams.L/quadParams.Jy;
b3=quadParams.L/quadParams.Jz;



% LEGEND
% x1=theta_x;
% x2=theta_x_dot;
% x3=theta_y;
% x4=theta_y_dot;
% x5=theta_z;
% x6=theta_z_dot;
% x7=z;
% x8=z_dot;






z1=x1_d-x1;
z3=x3_d-x3;
z5=x5_d-x5;

w2=(lincontroller.K2/2)^2*1/b1/2;
w3=(lincontroller.K3/2)^2*1/b2/2;
w4=(lincontroller.K4/2)^2*1/b3/2;


U_2_star=w2*z1;
U_3_star=w3*z3;
U_4_star=w4*z5;

== matlab function feedback_lin_p_with_noise_realistic/Subsystem/feedback_linearization_law ==
  data: x2 input; x4 input; x6 input; U_2_star input; U_2 output; U_3_star input; U_4_star input; U_3 output; U_4 output; lincontroller parameter; quadParams parameter
function [U_2,U_3,U_4] = feedback_linearization_law(x2,x4,x6,U_2_star,U_3_star,U_4_star,lincontroller,quadParams)


a1=(quadParams.Jy-quadParams.Jz)/quadParams.Jx;
a2=-quadParams.Jr/quadParams.Jx;
a3=(quadParams.Jz-quadParams.Jx)/quadParams.Jy;
a4=quadParams.Jr/quadParams.Jy;
a5=(quadParams.Jx-quadParams.Jy)/quadParams.Jz;
b1=quadParams.L/quadParams.Jx;
b2=quadParams.L/quadParams.Jy;
b3=quadParams.L/quadParams.Jz;



f_2 = 1/b1*(lincontroller.K2*x2-x4*x6*a1);
f_3 = 1/b2*(lincontroller.K3*x4-x2*x6*a3);
f_4 = 1/b3*(lincontroller.K4*x6-x4*x2*a5);


U_2 = f_2 + U_2_star;
U_3 = f_3 + U_3_star;
U_4 = f_4 + U_4_star;

== matlab function feedback_lin_p_with_noise_realistic/EKF_quadcopter1/CORRECTION ==
  data: x1k input; xkk output; Pkk output; x2k input; x3k input; x4k input; x5k input; x6k input; Pk input; z input
function [xkk,Pkk] = fcn(x1k,x2k,x3k,x4k,x5k,x6k,Pk,z)

% R = [2.782739102258347e-06 0 0 0 0 0;
%      0 1.936548166270313e-08 0 0 0 0;
%      0 0 2.718240466492716e-06 0 0 0;
%      0 0 0 1.809123162388460e-08 0 0;
%      0 0 0 0 5.587443411059212e-06 0;
%      0 0 0 0 0 5.587443411059212e-06];

R = [1.936548166270313e-08 0 0 0 0 0;
     0 2.782739102258347e-06 0 0 0 0;
     0 0 1.809123162388460e-08 0 0 0;
     0 0 0 2.718240466492716e-06 0 0;
     0 0 0 0 5.587443411059212e-06 0;
     0 0 0 0 0 2.976654513986432e-06];

H = [1 0 0 0 0 0;
     0 1 0 0 0 0;
     0 0 1 0 0 0;
     0 0 0 1 0 0;
     0 0 0 0 1 0;
     0 0 0 0 0 1];

xk = [x1k;x2k;x3k;x4k;x5k;x6k];

y = z - H * xk;

K = Pk*(H')/(H*Pk*(H') + R);

xkk = xk + K * y;
Pkk = (eye(6)-K * H) * Pk;

== matlab function feedback_lin_p_with_noise_realistic/EKF_quadcopter1/PROPAGATION ==
  data: x1 input; x1d output; x2 input; x3 input; x4 input; x5 input; x6 input; U_1 input; U_2 input; U_3 input; U_4 input; x2d output; x3d output; x4d output; x5d output; x6d output; Pk input; Pkp1 output
function [x1d,x2d,x3d,x4d,x5d,x6d,Pkp1] = fcn(x1,x2,x3,x4,x5,x6,U_1,U_2,U_3,U_4,Pk)

quadParams.g = 9.81;
quadParams.m = 1.07;
quadParams.Jx = 0.055;
quadParams.Jy = 0.055;
quadParams.Jz = 0.03;
quadParams.Jr=0;
quadParams.d = 0.1;
quadParams.L = 0.25;
quadParams.kd= 1.779e-07;  %Rotor torque coefficient(kg.m^2)   %M=kd*w^2
quadParams.kt = 1.105e-05;  %Rotor thrust coefficient(kg.m^2)  %T=kt*w^2

m = 1.07;
L = 0.25;
d = 0.055;
J = 0.055;
g = 9.81;
Ts = 0.002;

% Q = [0.0000000001 0 0 0 0 0;
%      0 0.00000001 0 0 0 0;
%      0 0 0.0000000001 0 0 0;
%      0 0 0 0.00000001 0 0;
%      0 0 0 0 0.0000000001 0;
%      0 0 0 0 0 0.00000001];

Q = [5e-16 0 0 0 0 0;
     0 1e-6 0 0 0 0;
     0 0 5e-16 0  0 0;
     0 0 0 1e-6 0 0;
     0 0 0 0 1e-13 0;
     0 0 0 0 0 5e-7];


a1=(quadParams.Jy-quadParams.Jz)/quadParams.Jx;
a2=-quadParams.Jr/quadParams.Jx;
a3=(quadParams.Jz-quadParams.Jx)/quadParams.Jy;
a4=quadParams.Jr/quadParams.Jy;
a5=(quadParams.Jx-quadParams.Jy)/quadParams.Jz;
b1=quadParams.L/quadParams.Jx;
b2=quadParams.L/quadParams.Jy;
b3=quadParams.L/quadParams.Jz;


x1d_dot =x2;

x2d_dot =x4*x6*a1 + b1*U_2;

x3d_dot =x4;

x4d_dot =x2*x6*a3+b2*U_3;

x5d_dot =x6;

x6d_dot =x4*x2*a5+b3*U_4;

x1d = x1 + x1d_dot*Ts;
x2d = x2 + x2d_dot*Ts;
x3d = x3 + x3d_dot*Ts;
x4d = x4 + x4d_dot*Ts;
x5d = x5 + x5d_dot*Ts;
x6d = x6 + x6d_dot*Ts;


F11 = 0;
F12 = 1;
F13 = 0;
F14 = 0;
F15 = 0;
F16 = 0;

F21 = 0;
F22 = 0;
F23 = 0;
F24 = x6*a1;
F25 = 0;
F26 = x4*a1;

F31 = 0;
F32 = 0;
F33 = 0;
F34 = 1;
F35 = 0;
F36 = 0;

F41 = 0;
F42 = x6*a3;
F43 = 0;
F44 = 0;
F45 = 0;
F46 = x2*a3;

F51 = 0;
F52 = 0;
F53 = 0;
F54 = 0;
F55 = 0;
F56 = 1;

F61 = 0;
F62 = x4*a5;
F63 = 0;
F64 = x2*a5;
F65 = 0;
F66 = 0;

F = [F11 F12 F13 F14 F15 F16;
     F21 F22 F23 F24 F25 F26;
     F31 F32 F33 F34 F35 F36;
     F41 F42 F43 F44 F45 F46;
     F51 F52 F53 F54 F55 F56;
     F61 F62 F63 F64 F65 F66];

PHI = expm(F * Ts);

Pkp1 = PHI * Pk * (PHI') + Q;

== matlab function feedback_lin_p_with_noise_realistic/Quadcopter Dynamics/Rigid Model/Rigid-Body Kinematic Model /Quaternion to rotation matrix ==
  data: q input; Reb output
function Reb = fcn(q)
%Function description;
%  The rotation matrix of the Aircraft-Body Coordinate Frame (ABCF) to the
%  Earth-Fixed Coordinate Frame (EFCF) is obtained from the quaternions
Reb = [q(1)*q(1) + q(2)*q(2) - q(3)*q(3) - q(4)*q(4), 2*(q(2)*q(3) - q(1)*q(4)), 2*(q(2)*q(4) + q(1)*q(3))
           2*(q(2)*q(3) + q(1)*q(4)), q(1)*q(1) - q(2)*q(2) + q(3)*q(3) - q(4)*q(4), 2*(q(3)*q(4) - q(1)*q(2))
           2*(q(2)*q(4) - q(1)*q(3)), 2*(q(3)*q(4) + q(1)*q(2)), q(1)*q(1) - q(2)*q(2) - q(3)*q(3) + q(4)*q(4)];
